simulink model "Model"  (R2024b)
settings: Solver=VariableStepAuto  StartTime=0.0  StopTime=500  FixedStep=Ts  RelTol=1e-3
values from neighbouring files (symbols this model uses):
  Ts = 1/fs    (= 0.0001)    [read_data.m]
undefined symbols (not defined in the file or in its folder): A, Ag, Ahims, Alqg, Alqg2, Alqg3, Ans, B, Bg, Bhims, Blqg, Blqg2, Blqg3, Bns, C, Cg, Chims, Clqg, Clqg2, Clqg3, Cns, D, Dg, Dhims, Dlqg, Dlqg2, Dlqg3, Dns, Tu, Ty
libraries: simulink x4
settings Model: Creator=yangshuyun  LastModifiedBy=yangshuyun

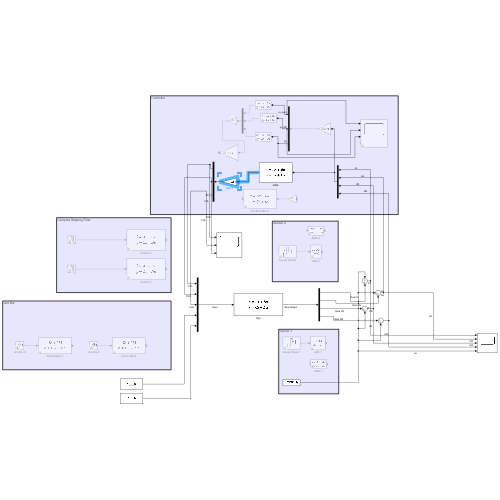
[thumbnail: Simulink's stored preview of the top-level diagram]
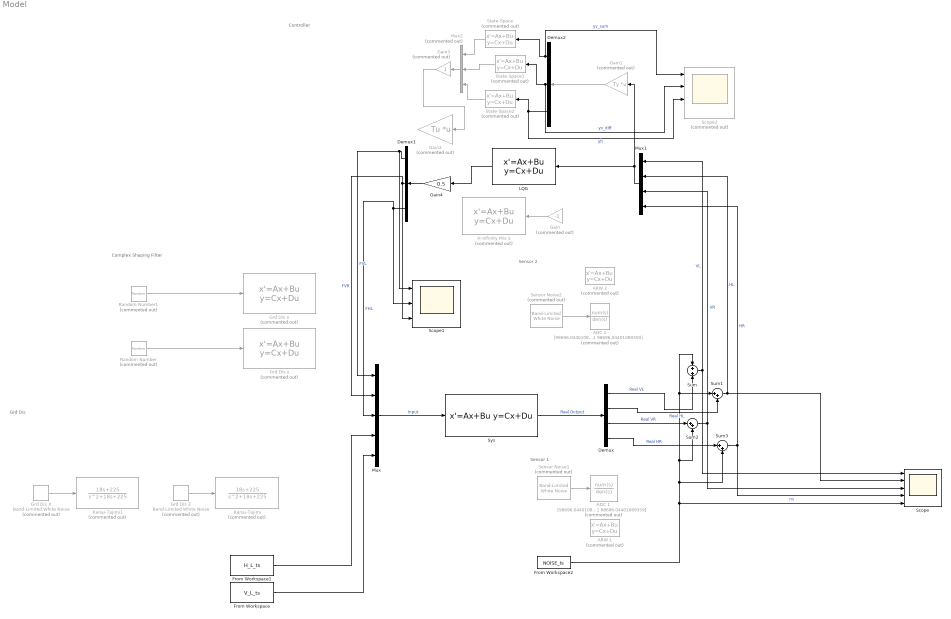
== system Model ==
  note: Controller
  note: Sensor 2
  note: Sensor 1
  note: Grd Dis
  note: Complex Shaping Filter
  ADC 1 : TransferFcn  Commented=on  Numerator=[98696.04401089359]  Denominator=[1 439.822971502571 98696.04401089359]
  ADC 2 : TransferFcn  Commented=on  Numerator=[98696.04401089359]  Denominator=[1 439.822971502571 98696.04401089359]
  ARW 1 : StateSpace  Commented=on  A=Ans  B=Bns  C=Cns  D=Dns  InitialCondition=0
  ARW 2 : StateSpace  Commented=on  A=Ans  B=Bns  C=Cns  D=Dns  InitialCondition=0
  Demux : Demux
  Demux1 : Demux  Outputs=3
  Demux2 : Demux  Outputs=3
  From Workspace : FromWorkspace  VariableName=V_L_ts  SampleTime=Ts
  From Workspace1 : FromWorkspace  VariableName=H_L_ts  SampleTime=Ts
  From Workspace2 : FromWorkspace  VariableName=NOISE_ts
  Gain : Gain  Commented=on  Gain=-1
  Gain1 : Gain  Commented=on  Gain=Ty  Multiplication=Matrix(K*u)
  Gain2 : Gain  Commented=on  Gain=Tu  Multiplication=Matrix(K*u)
  Gain3 : Gain  Commented=on
  Gain4 : Gain  Gain=0.5
  Grd Dis X : simulink/Sources/Band-Limited White Noise  Commented=on  Cov=[1e-14]  Ts=Ts  seed=[619]
  Grd Dis Z : simulink/Sources/Band-Limited White Noise  Commented=on  Cov=[1e-14]  Ts=Ts  seed=[42]
  Grd Dis x : StateSpace  Commented=on  A=Ag  B=Bg  C=Cg  D=Dg  InitialCondition=0
  Grd Dis z : StateSpace  Commented=on  A=Ag  B=Bg  C=Cg  D=Dg  InitialCondition=0
  H-Infinity Mix S : StateSpace  Commented=on  A=Ahims  B=Bhims  C=Chims  D=Dhims  InitialCondition=0
  Kanai-Tajimi : TransferFcn  Commented=on  Numerator=[18, 225]  Denominator=[1, 18, 225]
  Kanai-Tajimi1 : TransferFcn  Commented=on  Numerator=[18, 225]  Denominator=[1, 18, 225]
  LQG : StateSpace  A=Alqg  B=Blqg  C=Clqg  D=Dlqg  InitialCondition=0
  Mux : Mux  Inputs=5
  Mux1 : Mux
  Mux2 : Mux  Commented=on  Inputs=3
  Random Number : RandomNumber  Commented=on  Variance=100/Ts  Seed=42  SampleTime=Ts
  Random Number1 : RandomNumber  Commented=on  Variance=100/Ts  SampleTime=Ts
  Scope : Scope  NumInputPorts=5
  Scope1 : Scope  NumInputPorts=3
  Scope2 : Scope  Commented=on  NumInputPorts=4
  Sensor Noise1 : simulink/Sources/Band-Limited White Noise  Commented=on  Cov=1e-15  Ts=Ts  seed=[23341]
  Sensor Noise2 : simulink/Sources/Band-Limited White Noise  Commented=on  Cov=1e-15  Ts=Ts  seed=[114]
  State-Space : StateSpace  Commented=on  A=Alqg  B=Blqg  C=Clqg  D=Dlqg  InitialCondition=0
  State-Space1 : StateSpace  Commented=on  A=Alqg2  B=Blqg2  C=Clqg2  D=Dlqg2  InitialCondition=0
  State-Space2 : StateSpace  Commented=on  A=Alqg3  B=Blqg3  C=Clqg3  D=Dlqg3  InitialCondition=0
  Sum : Sum  Inputs=+|+
  Sum1 : Sum  Inputs=|++
  Sum2 : Sum  Inputs=|++
  Sum3 : Sum  Inputs=|++
  Sys : StateSpace  A=A  B=B  C=C  D=D  InitialCondition=0
  wires:
  Mux/1 -> Sys/1  "Input"
  Sys/1 -> Demux/1  "Real Output"
  Demux/4 -> Sum3/1  "Real HR"
  Demux/3 -> Sum2/1  "Real VR"
  Demux/2 -> Sum1/2  "Real HL"
  Demux/1 -> Sum/2  "Real VL"
  Demux1/1 -> Mux/1, Scope1/1  "FVL"
  Demux1/2 -> Mux/2, Scope1/3  "FVR"
  Demux1/3 -> Mux/3, Scope1/2  "FHL"
  Random Number1/1 -> Grd Dis x/1
  Random Number/1 -> Grd Dis z/1
  Sum/1 -> Mux1/1, Scope/1  "VL"
  Sum1/1 -> Scope/2, Mux1/2  "HL"
  Sum2/1 -> Scope/3, Mux1/3  "VR"
  Sum3/1 -> Scope/4, Mux1/4  "HR"
  Grd Dis Z/1 -> Kanai-Tajimi/1
  Grd Dis X/1 -> Kanai-Tajimi1/1
  Sensor Noise1/1 -> ADC 1/1
  Sensor Noise2/1 -> ADC 2/1
  Gain/1 -> H-Infinity Mix S/1
  State-Space/1 -> Mux2/1
  Demux2/1 -> Scope2/1, State-Space/1  "yv_sum"
  Demux2/3 -> State-Space2/1, Scope2/3  "yh"
  Mux2/1 -> Gain3/1
  State-Space2/1 -> Mux2/3
  Demux2/2 -> Scope2/2, State-Space1/1  "yv_diff"
  State-Space1/1 -> Mux2/2
  From Workspace1/1 -> Mux/4
  From Workspace/1 -> Mux/5
  Mux1/1 -> LQG/1, Gain1/1
  Gain1/1 -> Demux2/1
  Gain3/1 -> Gain2/1
  LQG/1 -> Gain4/1
  Gain4/1 -> Demux1/1
  From Workspace2/1 -> Scope/5, Sum1/1, Sum/1, Sum2/2, Sum3/2  "ns"
